simulink model "demo_ode"  (R2022a)
settings: Solver=VariableStepAuto  StartTime=0.0  StopTime=10.0  RelTol=1e-3
settings Model: Creator=gramschs  LastModifiedBy=gramschs

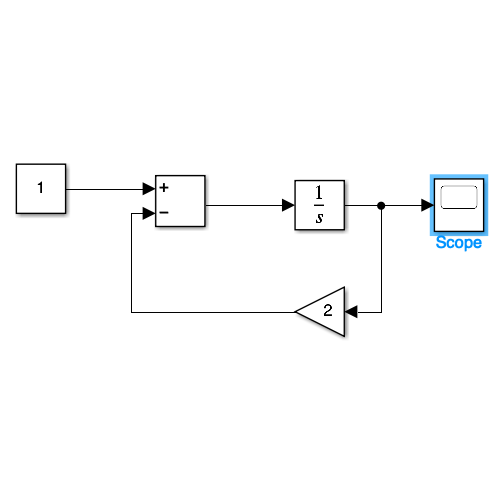
[thumbnail: Simulink's stored preview of the top-level diagram]
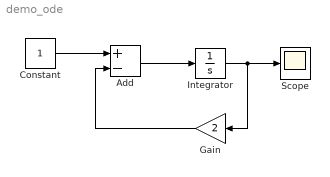
== system demo_ode ==
  Add : Sum  Inputs=+-
  Constant : Constant
  Gain : Gain  Gain=2
  Integrator : Integrator
  Scope : Scope
  wires:
  Constant/1 -> Add/1
  Add/1 -> Integrator/1
  Integrator/1 -> Gain/1, Scope/1
  Gain/1 -> Add/2
